simulink model "pid_control"  (R2022a)
settings: Solver=VariableStepAuto  StartTime=0.0  StopTime=30  RelTol=1e-3
values from neighbouring files (symbols this model uses):
  Kp = 0.80 * Kc    (= 2.36881775765)    [pid_relay.m]
  Td = 0.25 * Ti    (= 0.224)    [pid_relay.m]
  Ti = 0.64 * Tc    (= 0.896)    [pid_relay.m]
settings Model: Creator=josed  LastModifiedBy=josed

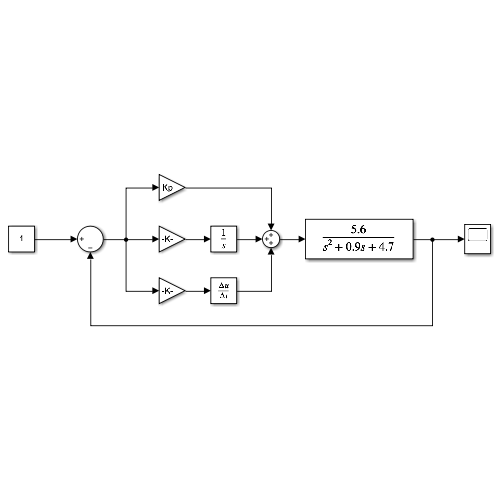
[thumbnail: Simulink's stored preview of the top-level diagram]
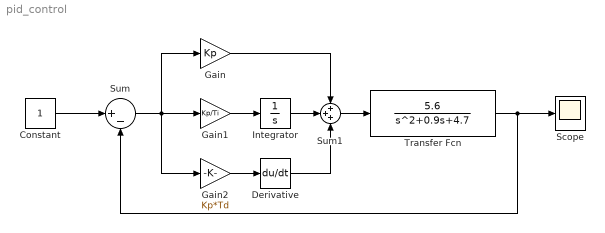
== system pid_control ==
  Constant : Constant
  Derivative : Derivative
  Gain : Gain  Gain=Kp
  Gain1 : Gain  Gain=Kp/Ti
  Gain2 : Gain  Gain=Kp*Td
  Integrator : Integrator
  Scope : Scope
  Sum : Sum  Inputs=|+-
  Sum1 : Sum  Inputs=+++
  Transfer Fcn : TransferFcn  Numerator=[5.6]  Denominator=[1 0.9 4.7]
  wires:
  Transfer Fcn/1 -> Scope/1, Sum/2
  Constant/1 -> Sum/1
  Sum1/1 -> Transfer Fcn/1
  Sum/1 -> Gain2/1, Gain/1, Gain1/1
  Gain/1 -> Sum1/1
  Gain1/1 -> Integrator/1
  Integrator/1 -> Sum1/2
  Gain2/1 -> Derivative/1
  Derivative/1 -> Sum1/3
